simulink model "simulate_2dof_robot"  (Simulink 7.7)
settings: Solver=ode45  StartTime=0.0  StopTime=10  FixedStep=0.01  MaxStep=0.001  MinStep=0.0005  RelTol=1e-3
undefined symbols (not defined in the file or in its folder): call_direct_dynamics_2dofplanar_fast, call_inverse_dynamics_2dofplanar_fast, call_third_order_planner
settings Model: Creator=arturo  LastModifiedBy=arturogilaparicio
settings DataIOCC: LimitDataPoints=off
settings DebuggingCC: StrictBusMsg=Warning

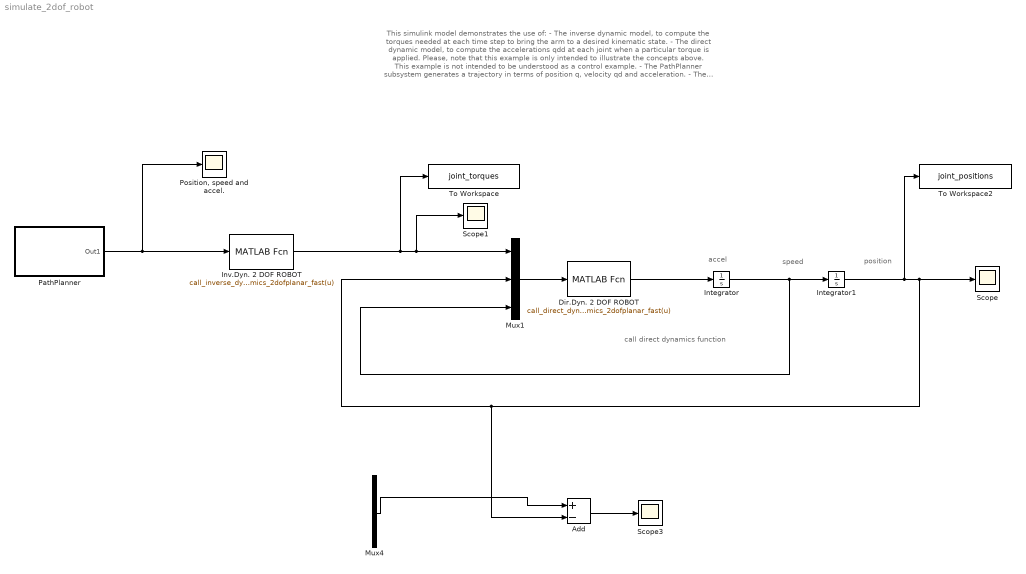
== system simulate_2dof_robot ==
  note: accel
  note: speed
  note: position
  note: This simulink model demonstrates the use of:
      | - The inverse dynamic model, to compute the torques needed at each time step to bring the arm to a desired kinematic state.
      | - The direct dynamic model, to compute the accelerations qdd at each joint when a particular torque is applied.
      | Please, note that this example is only intended to illustrate the concepts above. This example is not intended to be understood as
      | a control example.
      | - The PathPlanner subsystem generates a trajectory in terms of position q, velocity qd and acceleration.
      | - The example simulates a 2dof planar robot with two rotational joints.
      | - The planned q, qd and qdd are introduced in the inverse dynamic model. This block generates as output the torques needed at
      | each time step to bring the arm to the specified kinematic state.
      | - The joint torques are the introduced in the direct dynamics block. The inputs for this block are: the torques tau, the position and the
  note: call direct dynamics
      |  function
  Add : Sum  Inputs=+-
  Dir.Dyn. 2 DOF ROBOT : MATLABFcn  MATLABFcn=call_direct_dynamics_2dofplanar_fast(u)  OutputDimensions=2
  Integrator : Integrator  InitialCondition=[0 0]
  Integrator1 : Integrator  InitialCondition=[0 0]
  Inv.Dyn. 2 DOF ROBOT : MATLABFcn  MATLABFcn=call_inverse_dynamics_2dofplanar_fast(u)  OutputDimensions=2
  Mux1 : Mux  Inputs=3
  Mux4 : Mux  Inputs=2
  PathPlanner : Subsystem
      mask Display: port_label('output', 1, 'q, qd, qdd')
  "Position, speed and accel." : Scope
      settings: YMin=-0.05  YMax=0.525  SaveName=ScopeData2
  Scope : Scope
      settings: YMin=0.11  YMax=0.25
  Scope1 : Scope
      settings: YMin=4  YMax=20
  Scope3 : Scope
      settings: YMin=-1.2e-12  YMax=4e-13  SaveName=ScopeData3
  To Workspace : ToWorkspace  VariableName=joint_torques  SampleTime=-1  SaveFormat=Array
  To Workspace2 : ToWorkspace  VariableName=joint_positions  SampleTime=-1  SaveFormat=Array
  wires:
  Mux1/1 -> Dir.Dyn. 2 DOF ROBOT/1
  Dir.Dyn. 2 DOF ROBOT/1 -> Integrator/1
  Integrator/1 -> Integrator1/1, Mux1/3
  Integrator1/1 -> Scope/1, Add/2, Mux1/2, To Workspace2/1
  PathPlanner/1(Out1) -> Inv.Dyn. 2 DOF ROBOT/1, "Position, speed and accel."/1
  Mux4/1 -> Add/1
  Add/1 -> Scope3/1
  Inv.Dyn. 2 DOF ROBOT/1 -> To Workspace/1, Scope1/1, Mux1/1

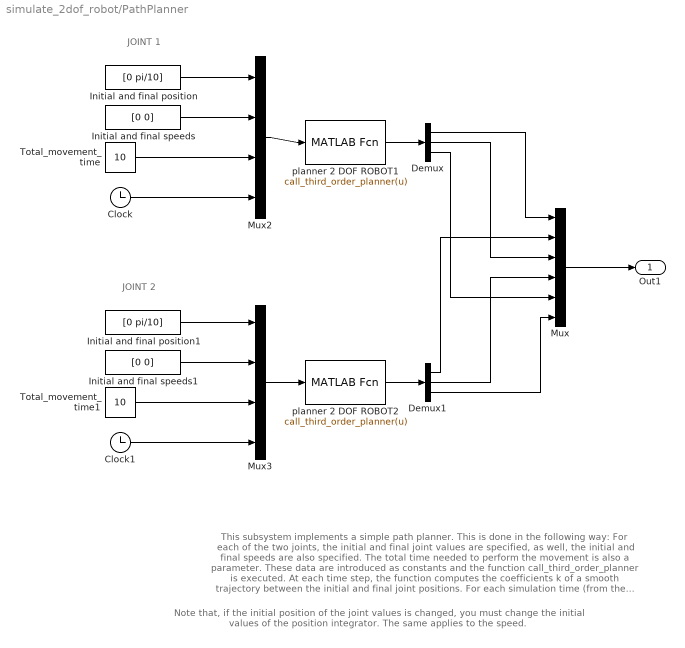
== system simulate_2dof_robot/PathPlanner ==
  note: JOINT 1
  note: JOINT 2
  note: This subsystem implements a simple path planner. This is done in the following way: For each of the two joints,
      | the initial and final joint values are specified, as well, the initial and final speeds are also specified. The total time needed to perform the movement is also
      | a parameter. These data are introduced as constants and the function call_third_order_planner is executed. At each time step, the function computes the coefficients
      | k of a smooth trajectory between the initial and final joint positions. For each simulation time (from the Clock source) que corresponding value for q(t), qd(t) and qdd(t) is computed.
      | The output is formed by 6 variables (2 values of position, 2 of joint speed and 2 of acceleration)
  note: Note that, if the initial position of the joint values is changed, you must change the initial values of the position integrator. The same applies to the speed.
  Clock : Clock
      settings: Decimation=10
  Clock1 : Clock
      settings: Decimation=10
  Demux : Demux  Outputs=3
  Demux1 : Demux  Outputs=3
  Initial and final position : Constant  Value=[0 pi/10]
  Initial and final position1 : Constant  Value=[0 pi/10]
  Initial and final speeds : Constant  Value=[0 0]
  Initial and final speeds1 : Constant  Value=[0 0]
  Mux : Mux  Inputs=6
  Mux2 : Mux
  Mux3 : Mux
  Total_movement_time : Constant  Value=10
  Total_movement_time1 : Constant  Value=10
  planner 2 DOF ROBOT1 : MATLABFcn  MATLABFcn=call_third_order_planner(u)  OutputDimensions=3
  planner 2 DOF ROBOT2 : MATLABFcn  MATLABFcn=call_third_order_planner(u)  OutputDimensions=3
  Out1 : Outport
  wires:
  Initial and final position/1 -> Mux2/1
  Initial and final speeds/1 -> Mux2/2
  Total_movement_time/1 -> Mux2/3
  Clock/1 -> Mux2/4
  Mux2/1 -> planner 2 DOF ROBOT1/1
  Initial and final position1/1 -> Mux3/1
  Initial and final speeds1/1 -> Mux3/2
  Total_movement_time1/1 -> Mux3/3
  Clock1/1 -> Mux3/4
  Mux3/1 -> planner 2 DOF ROBOT2/1
  planner 2 DOF ROBOT1/1 -> Demux/1
  planner 2 DOF ROBOT2/1 -> Demux1/1
  Demux/1 -> Mux/1
  Demux1/1 -> Mux/2
  Demux/2 -> Mux/3
  Demux1/2 -> Mux/4
  Demux/3 -> Mux/5
  Demux1/3 -> Mux/6
  Mux/1 -> Out1/1
